simulink library "library"  (R2021a)
settings: Solver=VariableStepAuto  StartTime=0.0  StopTime=10.0  RelTol=1e-3
values from neighbouring files (symbols this model uses):
  sensors = struct()    [setup.m]
  spacecraft = struct()    [setup.m]
undefined symbols (not defined in the file or in its folder): actuators, constants, control, observer, orbit
libraries: vrlib x14, $bdroot x5, cstblocks x1, simulink_extras x1
(part 1 of 2)
settings Model: Creator=loren  LastModifiedBy=loren
settings SolverCC: AlgebraicLoopSolver=TrustRegion
settings DebuggingCC: SFMachineParentedDataDiag=warning

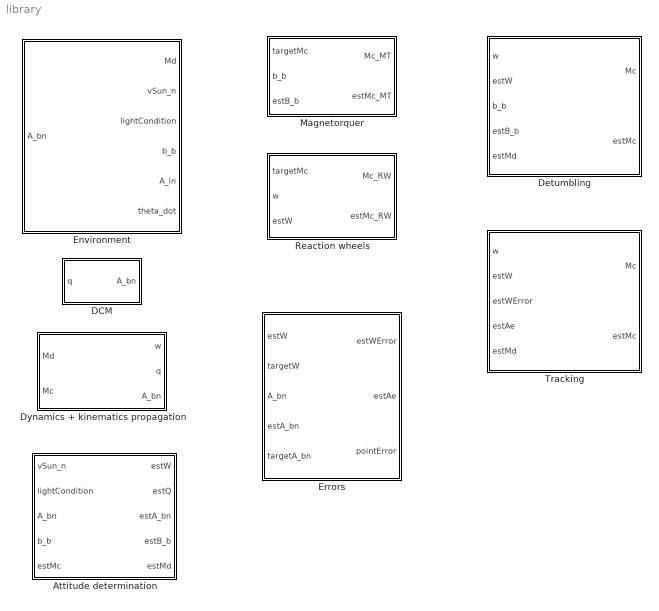
== system library ==
  Attitude determination : Subsystem
  DCM : Subsystem
  Detumbling : Subsystem
  Dynamics + kinematics propagation : Subsystem
  Environment : Subsystem
  Errors : Subsystem
  Magnetorquer : Subsystem
  Reaction wheels : Subsystem
  Tracking : Subsystem

== system library/Attitude determination ==
  vSun_n : Inport
  lightCondition : Inport  Port=2
  A_bn : Inport  Port=3
  b_b : Inport  Port=4
  estMc : Inport  Port=5
  Extended State Observer : Subsystem
  QUEST method : Subsystem
  Sensors : Subsystem
  estW : Outport
  estQ : Outport  Port=2
  estA_bn : Outport  Port=3
  estB_b : Outport  Port=4
  estMd : Outport  Port=5
  wires:
  Sensors/3(sunInSSFoV) -> QUEST method/3(sunInSSFoV)
  Sensors/2(v_n) -> QUEST method/2(v_n)
  Sensors/1(s_b) -> QUEST method/1(s_b)
  vSun_n/1 -> Sensors/1(vSun_n)
  lightCondition/1 -> Sensors/2(lightCondition)
  A_bn/1 -> Sensors/3(A_bn)
  b_b/1 -> Sensors/4(b_b)
  QUEST method/3(quatW) -> Extended State Observer/1(quatW)
  estMc/1 -> Extended State Observer/2(estMc)
  Extended State Observer/1(estW) -> estW/1
  Extended State Observer/2(estMd) -> estMd/1
  QUEST method/2(estA_bn) -> estA_bn/1
  QUEST method/1(estQ) -> estQ/1
  Sensors/4(estB_b) -> estB_b/1

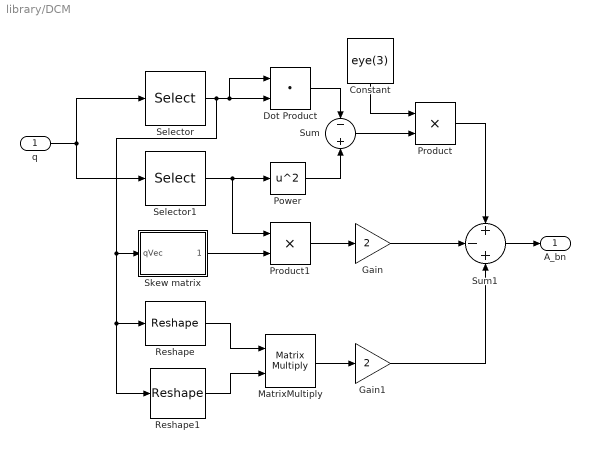
== system library/DCM ==
  q : Inport
  Constant : Constant  Value=eye(3)
  Dot Product : DotProduct  InputSameDT=on  OutDataTypeStr=Inherit: Inherit via internal rule
  Gain : Gain  Gain=2
  Gain1 : Gain  Gain=2
  MatrixMultiply : Product  Multiplication=Matrix(*)
  Power : Math  Operator=square  SaturateOnIntegerOverflow=on
  Product : Product
  Product1 : Product
  Reshape : Reshape  OutputDimensionality=Column vector (2-D)
  Reshape1 : Reshape  OutputDimensionality=Row vector (2-D)
  Selector : Selector  InputPortWidth=4  IndexOptions=Index vector (dialog)  Indices=[1 2 3]  OutputSizes=1
  Selector1 : Selector  InputPortWidth=4  IndexOptions=Index vector (dialog)  Indices=[4]  OutputSizes=1
  Skew matrix : Subsystem
  Sum : Sum  Inputs=-+
  Sum1 : Sum  Inputs=+-+
  A_bn : Outport
  wires:
  q/1 -> Selector/1, Selector1/1
  Selector/1 -> Reshape1/1, Reshape/1, Skew matrix/1(qVec), Dot Product/2, Dot Product/1
  Selector1/1 -> Product1/1, Power/1
  Power/1 -> Sum/2
  Dot Product/1 -> Sum/1
  Constant/1 -> Product/1
  Sum/1 -> Product/2
  Skew matrix/1(qWedge) -> Product1/2
  Product1/1 -> Gain/1
  Reshape/1 -> MatrixMultiply/1
  Reshape1/1 -> MatrixMultiply/2
  MatrixMultiply/1 -> Gain1/1
  Product/1 -> Sum1/1
  Gain/1 -> Sum1/2
  Gain1/1 -> Sum1/3
  Sum1/1 -> A_bn/1

== system library/Detumbling ==
  w : Inport
  estW : Inport  Port=2
  b_b : Inport  Port=3
  estB_b : Inport  Port=4
  estMd : Inport  Port=5
  Constant : Constant  Value=control.detumbling.SRD
  If : If  IfExpression=u1 == 1
  Merge : Merge
  Merge1 : Merge
  Proportional control (RWs) : Subsystem  TreatAsAtomicUnit=on
  Spin rate damping (MT) : Subsystem  TreatAsAtomicUnit=on
  Mc : Outport
  estMc : Outport  Port=2
  wires:
  Constant/1 -> If/1
  Proportional control (RWs)/2(estMc) -> Merge1/2
  Spin rate damping (MT)/2(estMc) -> Merge1/1
  Proportional control (RWs)/1(Mc) -> Merge/2
  Spin rate damping (MT)/1(Mc) -> Merge/1
  Merge/1 -> Mc/1
  Merge1/1 -> estMc/1
  w/1 -> Proportional control (RWs)/1(w)
  estW/1 -> Proportional control (RWs)/2(estW), Spin rate damping (MT)/1(estW)
  b_b/1 -> Spin rate damping (MT)/2(b_b)
  estB_b/1 -> Spin rate damping (MT)/3(estB_b)
  estMd/1 -> Proportional control (RWs)/3(estMd), Spin rate damping (MT)/4(estMd)
  If/1 -> Spin rate damping (MT)/Action
  If/2 -> Proportional control (RWs)/Action

== system library/Dynamics + kinematics propagation ==
  Md : Inport
  Mc : Inport  Port=2
  Euler equations : Subsystem
  Kinematics : Subsystem
  w : Outport
  q : Outport  Port=2
  A_bn : Outport  Port=3
  wires:
  Md/1 -> Euler equations/1(Md)
  Euler equations/1(w) -> w/1, Kinematics/1(w)
  Kinematics/1(q) -> q/1
  Kinematics/2(A_bn) -> A_bn/1
  Mc/1 -> Euler equations/2(Mc)

== system library/Environment ==
  A_bn : Inport
  Disturbances : Subsystem
  Orbit propagator : Subsystem
  Md : Outport
  vSun_n : Outport  Port=2
  lightCondition : Outport  Port=3
  b_b : Outport  Port=4
  A_ln : Outport  Port=5
  theta_dot : Outport  Port=6
  wires:
  A_bn/1 -> Orbit propagator/1(A_bn), Disturbances/1(A_bn)
  Orbit propagator/1(rrSc_n) -> Disturbances/2(rrSc_n)
  Orbit propagator/2(vvSc_n) -> Disturbances/3(vvSc_n)
  Orbit propagator/3(A_bl) -> Disturbances/4(A_bl)
  Disturbances/1(Md) -> Md/1
  Disturbances/2(vSun_n) -> vSun_n/1
  Disturbances/3(lightCondition) -> lightCondition/1
  Disturbances/4(b_b) -> b_b/1
  Orbit propagator/5(theta_dot) -> theta_dot/1
  Orbit propagator/4(A_ln) -> A_ln/1

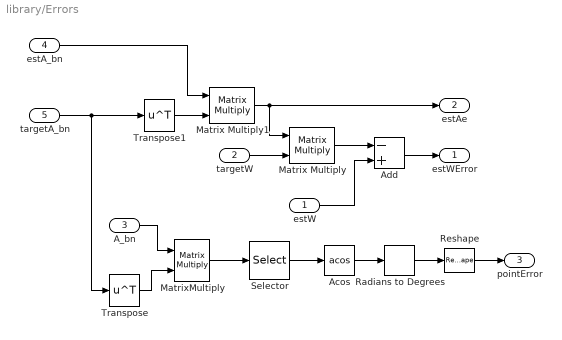
== system library/Errors ==
  estW : Inport
  targetW : Inport  Port=2
  A_bn : Inport  Port=3
  estA_bn : Inport  Port=4
  targetA_bn : Inport  Port=5
  Acos : Trigonometry  Operator=acos
  Add : Sum  Inputs=-+
  Matrix Multiply : Product  Multiplication=Matrix(*)
  Matrix Multiply1 : Product  Multiplication=Matrix(*)
  MatrixMultiply : Product  Multiplication=Matrix(*)
  Radians to Degrees : simulink_extras/Transformations/Radians to Degrees
  Reshape : Reshape
  Selector : Selector  NumberOfDimensions=2  InputPortWidth=3  IndexOptions=Index vector (dialog),Index vector (dialog)  Indices=1,1  OutputSizes=1,1
  Transpose : Math  Operator=transpose  SaturateOnIntegerOverflow=on
  Transpose1 : Math  Operator=transpose  SaturateOnIntegerOverflow=on
  estWError : Outport
  estAe : Outport  Port=2
  pointError : Outport  Port=3
  wires:
  targetW/1 -> Matrix Multiply/2
  targetA_bn/1 -> Transpose/1, Transpose1/1
  estA_bn/1 -> Matrix Multiply1/1
  Matrix Multiply1/1 -> Matrix Multiply/1, estAe/1
  Matrix Multiply/1 -> Add/1
  Acos/1 -> Radians to Degrees/1
  Radians to Degrees/1 -> Reshape/1
  estW/1 -> Add/2
  Add/1 -> estWError/1
  A_bn/1 -> MatrixMultiply/1
  Transpose/1 -> MatrixMultiply/2
  MatrixMultiply/1 -> Selector/1
  Selector/1 -> Acos/1
  Transpose1/1 -> Matrix Multiply1/2
  Reshape/1 -> pointError/1

== system library/Magnetorquer ==
  targetMc : Inport
  b_b : Inport  Port=2
  estB_b : Inport  Port=3
  Cross Product : vrlib/Utilities/Cross Product
  Cross Product1 : vrlib/Utilities/Cross Product
  Cross Product2 : vrlib/Utilities/Cross Product
  Divide : Product  Inputs=/*
  Dot Product : DotProduct  InputSameDT=on  OutDataTypeStr=Inherit: Inherit via internal rule
  Saturation : Saturate  UpperLimit=actuators.mt.D_max  LowerLimit=actuators.mt.D_min
  Mc_MT : Outport
  estMc_MT : Outport  Port=2
  wires:
  b_b/1 -> Cross Product1/2
  Cross Product2/1 -> estMc_MT/1
  Dot Product/1 -> Divide/1
  Cross Product1/1 -> Mc_MT/1
  Saturation/1 -> Cross Product2/1, Cross Product1/1
  targetMc/1 -> Cross Product/2
  Divide/1 -> Saturation/1
  Cross Product/1 -> Divide/2
  estB_b/1 -> Cross Product2/2, Dot Product/1, Dot Product/2, Cross Product/1

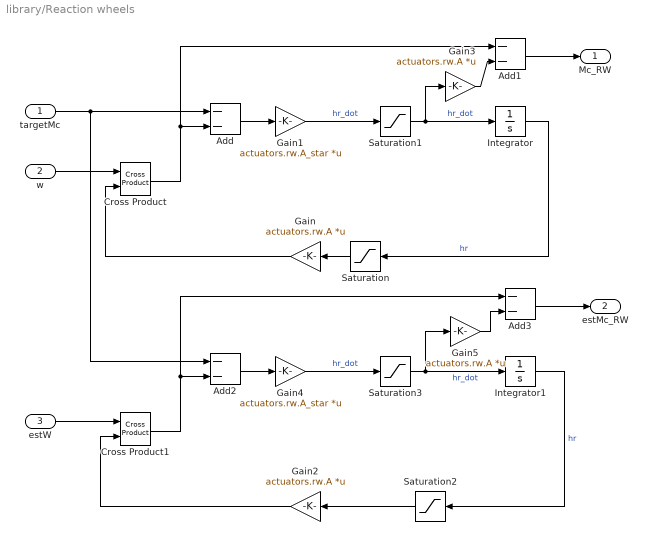
== system library/Reaction wheels ==
  targetMc : Inport
  w : Inport  Port=2
  estW : Inport  Port=3
  Add{,1..3} (4 alike) : Sum  Inputs=--
  Cross Product : vrlib/Utilities/Cross Product
  Cross Product1 : vrlib/Utilities/Cross Product
  Gain{,2..3,5} (4 alike) : Gain  Gain=actuators.rw.A  Multiplication=Matrix(K*u) (u vector)
  Gain1 : Gain  Gain=actuators.rw.A_star  Multiplication=Matrix(K*u) (u vector)
  Gain4 : Gain  Gain=actuators.rw.A_star  Multiplication=Matrix(K*u) (u vector)
  Integrator : Integrator  InitialCondition=actuators.rw.hr0
  Integrator1 : Integrator  InitialCondition=actuators.rw.hr0
  Saturation : Saturate  UpperLimit=actuators.rw.h_max  LowerLimit=-actuators.rw.h_max
  Saturation1 : Saturate  UpperLimit=actuators.rw.hdot_max  LowerLimit=-actuators.rw.hdot_max
  Saturation2 : Saturate  UpperLimit=actuators.rw.h_max  LowerLimit=-actuators.rw.h_max
  Saturation3 : Saturate  UpperLimit=actuators.rw.hdot_max  LowerLimit=-actuators.rw.hdot_max
  Mc_RW : Outport
  estMc_RW : Outport  Port=2
  wires:
  w/1 -> Cross Product/1
  Gain/1 -> Cross Product/2
  Cross Product/1 -> Add/2, Add1/1
  Gain1/1 -> Saturation1/1  "hr_dot"
  Integrator/1 -> Saturation/1  "hr"
  Saturation/1 -> Gain/1
  Add1/1 -> Mc_RW/1
  Add/1 -> Gain1/1
  Gain3/1 -> Add1/2
  Saturation1/1 -> Gain3/1, Integrator/1  "hr_dot"
  Gain5/1 -> Add3/2
  Add3/1 -> estMc_RW/1
  Add2/1 -> Gain4/1
  Saturation3/1 -> Integrator1/1, Gain5/1  "hr_dot"
  Cross Product1/1 -> Add2/2, Add3/1
  Integrator1/1 -> Saturation2/1  "hr"
  estW/1 -> Cross Product1/1
  targetMc/1 -> Add2/1, Add/1
  Saturation2/1 -> Gain2/1
  Gain2/1 -> Cross Product1/2
  Gain4/1 -> Saturation3/1  "hr_dot"

== system library/Tracking ==
  w : Inport
  estW : Inport  Port=2
  estWError : Inport  Port=3
  estAe : Inport  Port=4
  estMd : Inport  Port=5
  Ideal control law : Subsystem
  Reaction wheels : $bdroot/Reaction wheels  SystemSampleTime=-1  VariantActivationTime=update diagram  Latency=0  AutoFrameSizeCalculation=off
  Mc : Outport
  estMc : Outport  Port=2
  wires:
  w/1 -> Reaction wheels/2
  Ideal control law/1(Mc_id) -> Reaction wheels/1
  estW/1 -> Reaction wheels/3, Ideal control law/1(estW)
  estWError/1 -> Ideal control law/2(estWError)
  estAe/1 -> Ideal control law/3(estAe)
  estMd/1 -> Ideal control law/4(estMd)
  Reaction wheels/1 -> Mc/1
  Reaction wheels/2 -> estMc/1

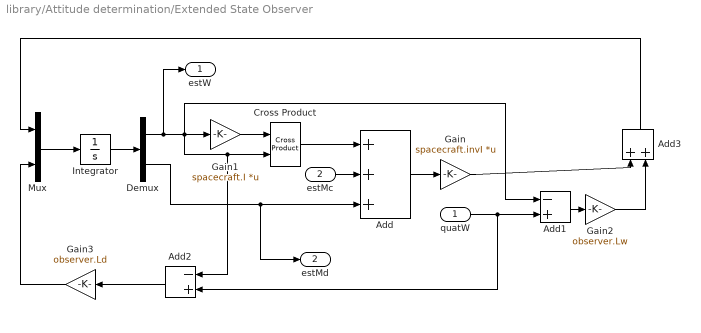
== system library/Attitude determination/Extended State Observer ==
  quatW : Inport
  estMc : Inport  Port=2
  Add : Sum  Inputs=+++
  Add1 : Sum  Inputs=-+
  Add2 : Sum  Inputs=-+
  Add3 : Sum
  Cross Product : vrlib/Utilities/Cross Product
  Demux : Demux  Outputs=[3, 3]
  Gain : Gain  Gain=spacecraft.invI  Multiplication=Matrix(K*u) (u vector)
  Gain1 : Gain  Gain=spacecraft.I  Multiplication=Matrix(K*u) (u vector)
  Gain2 : Gain  Gain=observer.Lw
  Gain3 : Gain  Gain=observer.Ld
  Integrator : Integrator  InitialCondition=[spacecraft.w0; observer.estMd0]
  Mux : Mux  Inputs=[3,3]
  estW : Outport
  estMd : Outport  Port=2
  wires:
  quatW/1 -> Add2/2, Add1/2
  Gain/1 -> Add3/1
  Demux/1 -> Add2/1, Cross Product/2, Add1/1, Gain1/1, estW/1
  Gain1/1 -> Cross Product/1
  Cross Product/1 -> Add/1
  estMc/1 -> Add/2
  Integrator/1 -> Demux/1
  Demux/2 -> estMd/1, Add/3
  Add/1 -> Gain/1
  Add1/1 -> Gain2/1
  Mux/1 -> Integrator/1
  Gain2/1 -> Add3/2
  Add2/1 -> Gain3/1
  Gain3/1 -> Mux/2
  Add3/1 -> Mux/1

== system library/Attitude determination/QUEST method ==
  s_b : Inport
  v_n : Inport  Port=2
  sunInSSFoV : Inport  Port=3
  Angular velocity estimation : Subsystem
  DCM : $bdroot/DCM  SystemSampleTime=-1  VariantActivationTime=update diagram  Latency=0  AutoFrameSizeCalculation=off
  MATLAB Function : MATLAB Function  TreatAsAtomicUnit=on
  Memory : Memory  InitialCondition=spacecraft.q0
  estQ : Outport
  estA_bn : Outport  Port=2
  quatW : Outport  Port=3
  wires:
  s_b/1 -> MATLAB Function/1(s_b)
  v_n/1 -> MATLAB Function/2(v_n)
  sunInSSFoV/1 -> MATLAB Function/3(sunInSSFoV)
  DCM/1 -> estA_bn/1
  Angular velocity estimation/1(quatW) -> quatW/1
  MATLAB Function/1(estQ) -> Memory/1, DCM/1, estQ/1, Angular velocity estimation/1(estQ)
  Memory/1 -> MATLAB Function/4(q_old)

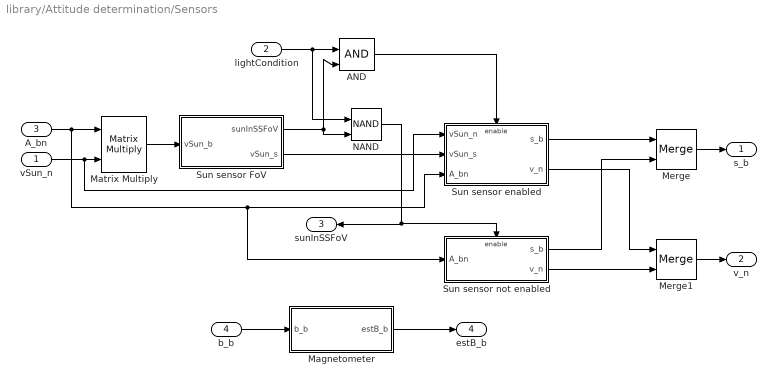
== system library/Attitude determination/Sensors ==
  vSun_n : Inport
  lightCondition : Inport  Port=2
  A_bn : Inport  Port=3
  b_b : Inport  Port=4
  AND : Logic  IconShape=distinctive  AllPortsSameDT=off  OutDataTypeStr=boolean
  Magnetometer : Subsystem
  Matrix Multiply : Product  Multiplication=Matrix(*)
  Merge : Merge
  Merge1 : Merge
  NAND : Logic  Operator=NAND  IconShape=distinctive  AllPortsSameDT=off  OutDataTypeStr=boolean
  Sun sensor FoV : Subsystem
  Sun sensor enabled : Subsystem  TreatAsAtomicUnit=on
  Sun sensor not enabled : Subsystem  TreatAsAtomicUnit=on
  s_b : Outport
  v_n : Outport  Port=2
  sunInSSFoV : Outport  Port=3
  estB_b : Outport  Port=4
  wires:
  Matrix Multiply/1 -> Sun sensor FoV/1(vSun_b)
  vSun_n/1 -> Sun sensor enabled/1(vSun_n), Matrix Multiply/2
  A_bn/1 -> Sun sensor not enabled/1(A_bn), Sun sensor enabled/3(A_bn), Matrix Multiply/1
  Merge/1 -> s_b/1
  Merge1/1 -> v_n/1
  b_b/1 -> Magnetometer/1(b_b)
  Magnetometer/1(estB_b) -> estB_b/1
  lightCondition/1 -> NAND/1, AND/1
  Sun sensor FoV/1(sunInSSFoV) -> AND/2, NAND/2
  AND/1 -> Sun sensor enabled/Enable
  NAND/1 -> sunInSSFoV/1, Sun sensor not enabled/Enable
  Sun sensor FoV/2(vSun_s) -> Sun sensor enabled/2(vSun_s)
  Sun sensor enabled/1(s_b) -> Merge/1
  Sun sensor not enabled/1(s_b) -> Merge/2
  Sun sensor enabled/2(v_n) -> Merge1/1
  Sun sensor not enabled/2(v_n) -> Merge1/2

== system library/DCM/Skew matrix ==
  qVec : Inport
  Constant : Constant  Value=0
  Constant1 : Constant  Value=0
  Constant2 : Constant  Value=0
  Demux : Demux  Outputs=3
  Gain : Gain  Gain=-1
  Gain1 : Gain  Gain=-1
  Gain2 : Gain  Gain=-1
  Matrix Concatenate : Concatenate  NumInputs=3  Mode=Multidimensional array
  Mux : Mux  Inputs=3
  Mux1 : Mux  Inputs=3
  Mux2 : Mux  Inputs=3
  Reshape : Reshape  OutputDimensionality=Row vector (2-D)
  Reshape1 : Reshape  OutputDimensionality=Row vector (2-D)
  Reshape2 : Reshape  OutputDimensionality=Row vector (2-D)
  qWedge : Outport
  wires:
  qVec/1 -> Demux/1
  Constant/1 -> Mux/1
  Gain/1 -> Mux/2
  Demux/3 -> Mux1/1, Gain/1
  Demux/2 -> Gain2/1, Mux/3
  Constant1/1 -> Mux1/2
  Gain1/1 -> Mux1/3
  Demux/1 -> Mux2/2, Gain1/1
  Constant2/1 -> Mux2/3
  Gain2/1 -> Mux2/1
  Mux1/1 -> Reshape1/1
  Mux/1 -> Reshape/1
  Mux2/1 -> Reshape2/1
  Matrix Concatenate/1 -> qWedge/1
  Reshape/1 -> Matrix Concatenate/1
  Reshape1/1 -> Matrix Concatenate/2
  Reshape2/1 -> Matrix Concatenate/3

== system library/Detumbling/Proportional control (RWs) ==
  w : Inport
  estW : Inport  Port=2
  estMd : Inport  Port=3
  Action Port : ActionPort
  Ideal control law : Subsystem  TreatAsAtomicUnit=on
  Reaction wheels : $bdroot/Reaction wheels  SystemSampleTime=-1  VariantActivationTime=update diagram  Latency=0  AutoFrameSizeCalculation=off
  Mc : Outport
  estMc : Outport  Port=2
  wires:
  Reaction wheels/1 -> Mc/1
  estMd/1 -> Ideal control law/2(estMd)
  estW/1 -> Ideal control law/1(estW), Reaction wheels/3
  w/1 -> Reaction wheels/2
  Ideal control law/1(Mc_id) -> Reaction wheels/1
  Reaction wheels/2 -> estMc/1

== system library/Detumbling/Spin rate damping (MT) ==
  estW : Inport
  b_b : Inport  Port=2
  estB_b : Inport  Port=3
  estMd : Inport  Port=4
  Action Port : ActionPort
  Ideal control law : Subsystem
  Magnetorquer : $bdroot/Magnetorquer  SystemSampleTime=-1  VariantActivationTime=update diagram  Latency=0  AutoFrameSizeCalculation=off
  Mc : Outport
  estMc : Outport  Port=2
  wires:
  Magnetorquer/2 -> estMc/1
  estW/1 -> Ideal control law/1(estW)
  estMd/1 -> Ideal control law/3(estMd)
  Magnetorquer/1 -> Mc/1
  Ideal control law/1(targetMc) -> Magnetorquer/1
  estB_b/1 -> Magnetorquer/3, Ideal control law/2(estB_b)
  b_b/1 -> Magnetorquer/2

== system library/Dynamics + kinematics propagation/Euler equations ==
  Md : Inport
  Mc : Inport  Port=2
  Add : Sum  Inputs=+++
  Cross Product : vrlib/Utilities/Cross Product
  Gain : Gain  Gain=spacecraft.I  Multiplication=Matrix(K*u) (u vector)
  Gain1 : Gain  Gain=spacecraft.invI  Multiplication=Matrix(K*u) (u vector)
  Integrator : Integrator  InitialCondition=spacecraft.w0
  w : Outport
  wires:
  Gain/1 -> Cross Product/1
  Integrator/1 -> w/1, Cross Product/2, Gain/1
  Cross Product/1 -> Add/1
  Gain1/1 -> Integrator/1
  Add/1 -> Gain1/1
  Md/1 -> Add/2
  Mc/1 -> Add/3

== system library/Dynamics + kinematics propagation/Kinematics ==
  w : Inport
  DCM : $bdroot/DCM  SystemSampleTime=-1  VariantActivationTime=update diagram  Latency=0  AutoFrameSizeCalculation=off
  Quaternion integration : Subsystem
  q : Outport
  A_bn : Outport  Port=2
  wires:
  w/1 -> Quaternion integration/1(w)
  Quaternion integration/1(q) -> DCM/1, q/1
  DCM/1 -> A_bn/1

== system library/Environment/Disturbances ==
  A_bn : Inport
  rrSc_n : Inport  Port=2
  vvSc_n : Inport  Port=3
  A_bl : Inport  Port=4
  Drag : Subsystem
  Earth magnetic field : Subsystem
  Gravity gradient : Subsystem
  Solar radiation pressure : Subsystem
      settings: PortSchema="{\"entries\":[{\"content\":{\"sides\":[{\"content\":{\"connectorIds\":[\"In1\",\"In2\"]},\"type\":\"ConnectorPlacement.EquallySpacedRectSide\",\"uuid\":\"1c58e148-737e-4c26-8467-bf4a1427bac3\"},{\"content\":{\"connectorIds\":[\"Out1\"],\"side\":\"RIGHT\"},\"type\":\"ConnectorPlacement.EquallySpacedRectSide\",\"uuid\":\"1132a1c1-392d-4550-8b40-4ae647f3a6c1\"},{\"content\":{\"connectorIds\":[\"Out2\",\"Out3\"],\"side\":\"TOP\"},\"type\":\"ConnectorPlacement.EquallySpacedRectSide\",\"uuid\":\"8cec875a-7b2b-408d-843f-f50e353248f2\"},{\"content\":{\"connectorIds\":[],\"side\":\"HIDDEN\"},\"type\":\"ConnectorPlacement.EquallySpacedRectSide\",\"uuid\":\"95559ba3-4215-4144-a5e7-008848b1ca72\"}]},\"type\":\"ConnectorPlacement.EquallySpacedConnector\",\"uuid\":\"cb15f690-b6d7-424c-84c7-df23a46a4e4f\"}],\"packageUris\":[\"http://schema.mathworks.com/mf0/Connector/R2020b\"],\"version\":\"1.0\"}"
  Sum : Sum  Inputs=++++
  Md : Outport
  vSun_n : Outport  Port=2
  lightCondition : Outport  Port=3
  b_b : Outport  Port=4
  wires:
  Solar radiation pressure/1(M_srp) -> Sum/1
  A_bn/1 -> Solar radiation pressure/2(A_bn), Drag/3(A_bn), Earth magnetic field/2(A_bn)
  vvSc_n/1 -> Drag/2(vvSc_n)
  rrSc_n/1 -> Gravity gradient/1(rrSc_n), Drag/1(rrSc_n), Earth magnetic field/1(rrSc_n), Solar radiation pressure/1(rrSc_n)
  Gravity gradient/1(M_gg) -> Sum/3
  Drag/1(M_drag) -> Sum/4
  Earth magnetic field/2(M_b) -> Sum/2
  Sum/1 -> Md/1
  A_bl/1 -> Gravity gradient/2(A_bl)
  Solar radiation pressure/2(vSun_n) -> vSun_n/1
  Solar radiation pressure/3(lightCondition) -> lightCondition/1
  Earth magnetic field/1(b_b) -> b_b/1

== system library/Environment/Orbit propagator ==
  A_bn : Inport
  Integrator1 : Integrator  InitialCondition=orbit.theta0
  LVLH frame : Subsystem
  Position and velocity (inertial frame) : Subsystem
  True anomaly ODE : Subsystem
  rrSc_n : Outport
  vvSc_n : Outport  Port=2
  A_bl : Outport  Port=3
  A_ln : Outport  Port=4
  theta_dot : Outport  Port=5
  wires:
  True anomaly ODE/1(theta_dot) -> Integrator1/1, theta_dot/1
  Integrator1/1 -> LVLH frame/1(theta), True anomaly ODE/1(theta), Position and velocity (inertial frame)/1(theta)
  Position and velocity (inertial frame)/1(rrSc_n) -> rrSc_n/1
  Position and velocity (inertial frame)/2(vvSc_n) -> vvSc_n/1
  LVLH frame/1(A_bl) -> A_bl/1
  A_bn/1 -> LVLH frame/2(A_bn)
  LVLH frame/2(A_ln) -> A_ln/1

== system library/Tracking/Ideal control law ==
  estW : Inport
  estWError : Inport  Port=2
  estAe : Inport  Port=3
  estMd : Inport  Port=4
  Add : Sum  Inputs=--+-
  Cross Product : vrlib/Utilities/Cross Product
  Gain : Gain  Gain=control.tracking.kw
  Gain1 : Gain  Gain=control.tracking.kae
  Gain3 : Gain  Gain=spacecraft.I  Multiplication=Matrix(K*u) (u vector)
  MATLAB Function : MATLAB Function  TreatAsAtomicUnit=on
  Mc_id : Outport
  wires:
  Add/1 -> Mc_id/1
  MATLAB Function/1(lf) -> Gain1/1
  estAe/1 -> MATLAB Function/1(estAe)
  Gain/1 -> Add/1
  Gain3/1 -> Cross Product/2
  estMd/1 -> Add/4
  Gain1/1 -> Add/2
  estWError/1 -> Gain/1
  estW/1 -> Gain3/1, Cross Product/1
  Cross Product/1 -> Add/3

== system library/Attitude determination/QUEST method/Angular velocity estimation ==
  estQ : Inport
  Constant : Constant
  Derivative : Derivative  CoefficientInTFapproximation=1/10
  Gain : Gain  Gain=2
  Matrix Multiply : Product  Multiplication=Matrix(*)
  Quaternion matrix : Subsystem
  Varying Lowpass Filter : cstblocks/Linear Parameter Varying/Varying Lowpass Filter  N=1
  quatW : Outport
  wires:
  Derivative/1 -> Matrix Multiply/2  "dotQest"
  Matrix Multiply/1 -> Gain/1
  Gain/1 -> quatW/1
  estQ/1 -> Quaternion matrix/1(q), Varying Lowpass Filter/1
  Varying Lowpass Filter/1 -> Derivative/1
  Constant/1 -> Varying Lowpass Filter/2
  Quaternion matrix/1(Q_star) -> Matrix Multiply/1

== system library/Attitude determination/Sensors/Magnetometer ==
  b_b : Inport
  Add : Sum
  MATLAB Function : MATLAB Function  TreatAsAtomicUnit=on
  Matrix Multiply : Product  Multiplication=Matrix(*)
  Random Number : RandomNumber  Variance=sensors.mm.sigmaPhi^2  Seed=randi(1e5, 1, 1)  SampleTime=sensors.mm.Ts
  Random Number1 : RandomNumber  Variance=sensors.mm.sigmaTheta^2  Seed=randi(1e5, 1, 1)  SampleTime=sensors.mm.Ts
  Random Number2 : RandomNumber  Variance=sensors.mm.sigmaPsi^2  Seed=randi(1e5, 1, 1)  SampleTime=sensors.mm.Ts
  Random Number3 : RandomNumber  Variance=sensors.mm.eps^2*ones(3,1)  Seed=randi(1e5, 1, 1)  SampleTime=sensors.mm.Ts
  Zero-Order Hold : ZeroOrderHold  SampleTime=sensors.mm.Ts
  estB_b : Outport
  wires:
  b_b/1 -> Zero-Order Hold/1
  Random Number/1 -> MATLAB Function/1(phi)
  Random Number1/1 -> MATLAB Function/2(theta)
  Random Number2/1 -> MATLAB Function/3(psi)
  Zero-Order Hold/1 -> Add/1
  MATLAB Function/1(A_err) -> Matrix Multiply/1
  Matrix Multiply/1 -> estB_b/1
  Add/1 -> Matrix Multiply/2
  Random Number3/1 -> Add/2

== system library/Attitude determination/Sensors/Sun sensor FoV ==
  vSun_b : Inport
  Acos : Trigonometry  Operator=acos
  Constant : Constant  Value=sensors.ss.FoV
  Constant2 : Constant  Value=[1; 0; 0]
  Dot Product : DotProduct  InputSameDT=on  OutDataTypeStr=Inherit: Inherit via internal rule
  Gain : Gain  Gain=sensors.ss.A_sb  Multiplication=Matrix(K*u) (u vector)
  Less Than : RelationalOperator  Operator=<  OutDataTypeStr=boolean  RndMeth=Simplest
  sunInSSFoV : Outport
  vSun_s : Outport  Port=2
  wires:
  Less Than/1 -> sunInSSFoV/1
  Constant/1 -> Less Than/2
  Acos/1 -> Less Than/1
  Dot Product/1 -> Acos/1
  vSun_b/1 -> Gain/1
  Gain/1 -> Dot Product/2, vSun_s/1
  Constant2/1 -> Dot Product/1

== system library/Attitude determination/Sensors/Sun sensor enabled ==
  vSun_n : Inport
  vSun_s : Inport  Port=2
  A_bn : Inport  Port=3
  Enable : EnablePort
  Matrix Concatenate : Concatenate  Mode=Multidimensional array  ConcatenateDimension=2
  Matrix Concatenate1 : Concatenate  Mode=Multidimensional array  ConcatenateDimension=2
  Star tracker : Subsystem
  Sun sensor : Subsystem
  Zero-Order Hold : ZeroOrderHold  SampleTime=max([sensors.ss.Ts, sensors.st.Ts])
  s_b : Outport
  v_n : Outport  Port=2
  wires:
  vSun_s/1 -> Sun sensor/1(vSun_s)
  A_bn/1 -> Star tracker/1(A_bn)
  Sun sensor/1(sSun_b) -> Matrix Concatenate/1
  Star tracker/1(sStars_b) -> Matrix Concatenate/2
  Star tracker/2(vStars_n) -> Matrix Concatenate1/2
  vSun_n/1 -> Zero-Order Hold/1
  Matrix Concatenate/1 -> s_b/1
  Matrix Concatenate1/1 -> v_n/1
  Zero-Order Hold/1 -> Matrix Concatenate1/1

== system library/Attitude determination/Sensors/Sun sensor not enabled ==
  A_bn : Inport
  Enable : EnablePort
  Star tracker : Subsystem
  s_b : Outport
  v_n : Outport  Port=2
  wires:
  Star tracker/1(sStars_b) -> s_b/1
  Star tracker/2(vStars_n) -> v_n/1
  A_bn/1 -> Star tracker/1(A_bn)

== system library/Detumbling/Proportional control (RWs)/Ideal control law ==
  estW : Inport
  estMd : Inport  Port=2
  Add : Sum  Inputs=+-
  Gain : Gain  Gain=-control.detumbling.kp
  Mc_id : Outport
  wires:
  estMd/1 -> Add/2
  Add/1 -> Mc_id/1
  Gain/1 -> Add/1
  estW/1 -> Gain/1

== system library/Detumbling/Spin rate damping (MT)/Ideal control law ==
  estW : Inport
  estB_b : Inport  Port=2
  estMd : Inport  Port=3
  Add : Sum  Inputs=+-
  Cross Product : vrlib/Utilities/Cross Product
  Cross Product1 : vrlib/Utilities/Cross Product
  Gain : Gain  Gain=-control.detumbling.kb
  targetMc : Outport
  wires:
  Cross Product1/1 -> Add/1
  Gain/1 -> Cross Product1/1
  estW/1 -> Cross Product/2
  estB_b/1 -> Cross Product1/2, Cross Product/1
  Cross Product/1 -> Gain/1
  Add/1 -> targetMc/1
  estMd/1 -> Add/2

== system library/Dynamics + kinematics propagation/Kinematics/Quaternion integration ==
  w : Inport
  Gain : Gain  Gain=1/2
  Integrator : Integrator  InitialCondition=spacecraft.q0
  MatrixMultiply : Product  Multiplication=Matrix(*)
  Normalize Vector : vrlib/Utilities/Normalize Vector  maxzero=0
  Omega matrix : Subsystem
  q : Outport
  wires:
  Integrator/1 -> Normalize Vector/1
  Normalize Vector/1 -> q/1, MatrixMultiply/2
  Omega matrix/1(OM_mat) -> MatrixMultiply/1
  MatrixMultiply/1 -> Gain/1
  Gain/1 -> Integrator/1
  w/1 -> Omega matrix/1(w)

== system library/Environment/Disturbances/Drag ==
  rrSc_n : Inport
  vvSc_n : Inport  Port=2
  A_bn : Inport  Port=3
  Constant : Constant  Value=constants.rho
  MATLAB Function : MATLAB Function  TreatAsAtomicUnit=on
  M_drag : Outport
  wires:
  rrSc_n/1 -> MATLAB Function/1(rrSc_n)
  MATLAB Function/1(mDrag) -> M_drag/1
  vvSc_n/1 -> MATLAB Function/2(vvSc_n)
  A_bn/1 -> MATLAB Function/3(A_bn)
  Constant/1 -> MATLAB Function/4(rho)

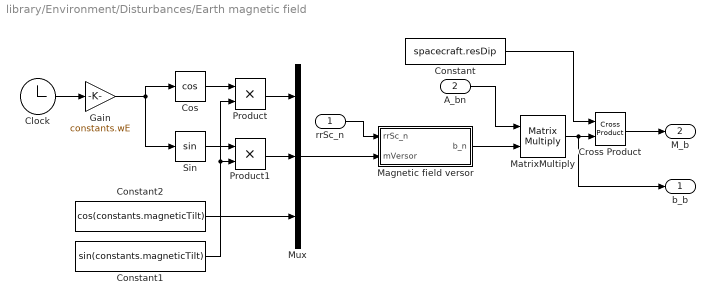
== system library/Environment/Disturbances/Earth magnetic field ==
  rrSc_n : Inport
  A_bn : Inport  Port=2
  Clock : Clock
  Constant : Constant  Value=spacecraft.resDip
  Constant1 : Constant  Value=sin(constants.magneticTilt)
  Constant2 : Constant  Value=cos(constants.magneticTilt)
  Cos : Trigonometry  Operator=cos
  Cross Product : vrlib/Utilities/Cross Product
  Gain : Gain  Gain=constants.wE
  Magnetic field versor : Subsystem
  MatrixMultiply : Product  Multiplication=Matrix(*)
  Mux : Mux  Inputs=3
  Product : Product
  Product1 : Product
  Sin : Trigonometry
  b_b : Outport
  M_b : Outport  Port=2
  wires:
  Clock/1 -> Gain/1
  Constant/1 -> Cross Product/1
  Gain/1 -> Sin/1, Cos/1
  Constant2/1 -> Mux/3
  Sin/1 -> Product1/1
  Cos/1 -> Product/1
  Product/1 -> Mux/1
  Product1/1 -> Mux/2
  Constant1/1 -> Product/2, Product1/2
  A_bn/1 -> MatrixMultiply/1
  rrSc_n/1 -> Magnetic field versor/1(rrSc_n)
  Mux/1 -> Magnetic field versor/2(mVersor)
  Magnetic field versor/1(b_n) -> MatrixMultiply/2
  MatrixMultiply/1 -> b_b/1, Cross Product/2
  Cross Product/1 -> M_b/1

== system library/Environment/Disturbances/Gravity gradient ==
  rrSc_n : Inport
  A_bl : Inport  Port=2
  Constant : Constant  Value=[1 0 0]
  Gravity gradient : Subsystem
  MatrixMultiply : Product  Multiplication=Matrix(*)
  M_gg : Outport
  wires:
  Constant/1 -> MatrixMultiply/2
  MatrixMultiply/1 -> Gravity gradient/2(c)  "c"
  A_bl/1 -> MatrixMultiply/1
  Gravity gradient/1(M_gg) -> M_gg/1
  rrSc_n/1 -> Gravity gradient/1(rrSc_n)

== system library/Environment/Disturbances/Solar radiation pressure ==
  note: Determine whether the s/c is in sunlight or not
  rrSc_n : Inport
  A_bn : Inport  Port=2
  If : If  IfExpression=u1 == 1
  Merge : Merge
  SRP: active : Subsystem  TreatAsAtomicUnit=on
  SRP: non-active : Subsystem  TreatAsAtomicUnit=on
  Shadow cone of the Earth : Subsystem
  Sun position in the Earth inertial frame : Subsystem
  M_srp : Outport
  vSun_n : Outport  Port=2
  lightCondition : Outport  Port=3
  wires:
  Shadow cone of the Earth/1(lightCondition) -> lightCondition/1, If/1
  If/2 -> SRP: non-active/Action
  If/1 -> SRP: active/Action
  SRP: non-active/1(mSRP) -> Merge/2
  rrSc_n/1 -> SRP: active/1(rrSc_n), Shadow cone of the Earth/1(rrSc_n)
  Merge/1 -> M_srp/1
  SRP: active/1(mSRP) -> Merge/1
  Sun position in the Earth inertial frame/1(rrSun_n) -> SRP: active/2(rrSun_n), Shadow cone of the Earth/2(rrSun_n)
  SRP: active/2(vSun_n) -> vSun_n/1
  A_bn/1 -> SRP: active/3(A_bn)

== system library/Environment/Orbit propagator/LVLH frame ==
  theta : Inport
  A_bn : Inport  Port=2
  LVLH to inclined orbit frame : Subsystem
  Product : Product  Multiplication=Matrix(*)
  Product1 : Product  Multiplication=Matrix(*)
  R1(i) : Constant  Value=[1 0 0; 0 cos(orbit.i) sin(orbit.i); 0 -sin(orbit.i) cos(orbit.i)];
  Transpose : Math  Operator=transpose  SaturateOnIntegerOverflow=on
  A_bl : Outport
  A_ln : Outport  Port=2
  wires:
  Transpose/1 -> Product1/2  "A_nl"
  Product/1 -> A_ln/1, Transpose/1
  A_bn/1 -> Product1/1
  Product1/1 -> A_bl/1  "A_bl"
  R1(i)/1 -> Product/2
  theta/1 -> LVLH to inclined orbit frame/1(theta)
  LVLH to inclined orbit frame/1(A_li) -> Product/1

== system library/Environment/Orbit propagator/Position and velocity (inertial frame) ==
  theta : Inport
  Matrix Multiply : Product  Multiplication=Matrix(*)
  Matrix Multiply1 : Product  Multiplication=Matrix(*)
  Position and velocity (perifocal frame) : Subsystem
  R1(i) : Constant  Value=[1 0 0; 0 cos(orbit.i) sin(orbit.i); 0 -sin(orbit.i) cos(orbit.i)];
  R3(OM) : Constant  Value=[cos(orbit.OM), sin(orbit.OM), 0; -sin(orbit.OM), cos(orbit.OM), 0; 0, 0, 1]
  R3(om) : Constant  Value=[cos(orbit.om), sin(orbit.om), 0; -sin(orbit.om), cos(orbit.om), 0; 0, 0, 1]
  Rotation matrix (perifocal-inertial) : Product  Inputs=3  Multiplication=Matrix(*)
  Transpose : Math  Operator=transpose  SaturateOnIntegerOverflow=on
  rrSc_n : Outport
  vvSc_n : Outport  Port=2
  wires:
  Matrix Multiply/1 -> rrSc_n/1
  Position and velocity (perifocal frame)/2(vvSc_pf) -> Matrix Multiply1/2
  Matrix Multiply1/1 -> vvSc_n/1
  R3(om)/1 -> Rotation matrix (perifocal-inertial)/1
  R1(i)/1 -> Rotation matrix (perifocal-inertial)/2
  Rotation matrix (perifocal-inertial)/1 -> Transpose/1
  Transpose/1 -> Matrix Multiply1/1, Matrix Multiply/1
  R3(OM)/1 -> Rotation matrix (perifocal-inertial)/3
  Position and velocity (perifocal frame)/1(rrSc_pf) -> Matrix Multiply/2
  theta/1 -> Position and velocity (perifocal frame)/1(theta)

== system library/Environment/Orbit propagator/True anomaly ODE ==
  theta : Inport
  Add : Sum
  Constant1 : Constant
  Cos : Trigonometry  Operator=cos
  Gain : Gain  Gain=sqrt(constants.mu/orbit.a^3)
  Gain1 : Gain  Gain=(1 - orbit.e^2)^(-3/2)
  Gain2 : Gain  Gain=orbit.e
  Power : Math  Operator=square  SaturateOnIntegerOverflow=on
  theta_dot : Outport
  wires:
  theta/1 -> Cos/1
  Constant1/1 -> Add/1
  Cos/1 -> Gain2/1
  Gain2/1 -> Add/2
  Add/1 -> Power/1
  Power/1 -> Gain/1
  Gain/1 -> Gain1/1
  Gain1/1 -> theta_dot/1

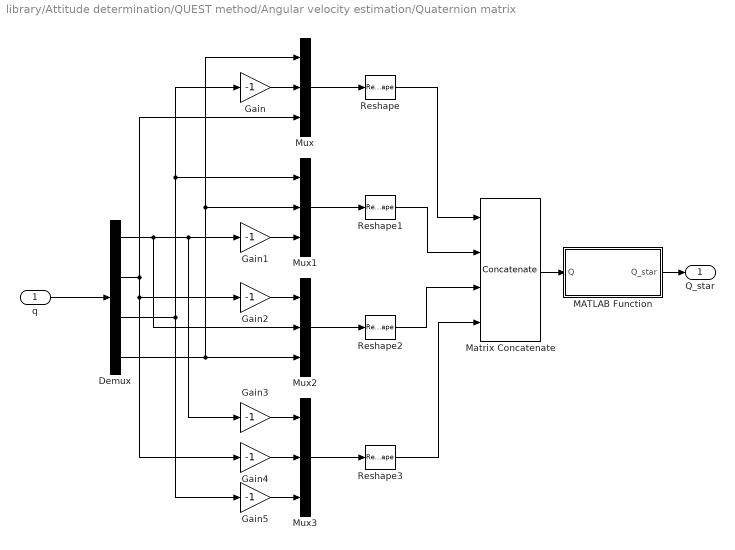
== system library/Attitude determination/QUEST method/Angular velocity estimation/Quaternion matrix ==
  q : Inport
  Demux : Demux
  Gain{,1..5} (6 alike) : Gain  Gain=-1
  MATLAB Function : MATLAB Function  TreatAsAtomicUnit=on
  Matrix Concatenate : Concatenate  NumInputs=4  Mode=Multidimensional array
  Mux{,1..3} (4 alike) : Mux  Inputs=3
  Reshape{,1..3} (4 alike) : Reshape  OutputDimensionality=Row vector (2-D)
  Q_star : Outport
  wires:
  q/1 -> Demux/1
  Demux/4 -> Mux1/2, Mux/1, Mux2/3
  Gain/1 -> Mux/2
  Demux/3 -> Gain5/1, Mux1/1, Gain/1
  Demux/2 -> Gain2/1, Gain4/1, Mux/3
  Gain1/1 -> Mux1/3
  Demux/1 -> Mux2/2, Gain3/1, Gain1/1
  Gain2/1 -> Mux2/1
  Gain3/1 -> Mux3/1
  Gain4/1 -> Mux3/2
  Gain5/1 -> Mux3/3
  Mux3/1 -> Reshape3/1
  Mux2/1 -> Reshape2/1
  Mux1/1 -> Reshape1/1
  Mux/1 -> Reshape/1
  Reshape/1 -> Matrix Concatenate/1
  Reshape1/1 -> Matrix Concatenate/2
  Reshape2/1 -> Matrix Concatenate/3
  Reshape3/1 -> Matrix Concatenate/4
  Matrix Concatenate/1 -> MATLAB Function/1(Q)
  MATLAB Function/1(Q_star) -> Q_star/1

== system library/Attitude determination/Sensors/Sun sensor enabled/Star tracker ==
  A_bn : Inport
  MATLAB Function : MATLAB Function  TreatAsAtomicUnit=on
  Memory : Memory  InitialCondition=sensors.st.vStars_n_init(:,2:end)  InheritSampleTime=on  LinearizeMemory=on
  Random Number : RandomNumber  Variance=sensors.st.sigmaPhi^2  Seed=randi(1e5,1,1)  SampleTime=max([sensors.ss.Ts, sensors.st.Ts])
  Random Number1 : RandomNumber  Variance=sensors.st.sigmaTheta^2  Seed=randi(1e5,1,1)  SampleTime=max([sensors.ss.Ts, sensors.st.Ts])
  Random Number2 : RandomNumber  Variance=sensors.st.sigmaPsi^2  Seed=randi(1e5,1,1)  SampleTime=max([sensors.ss.Ts, sensors.st.Ts])
  Zero-Order Hold : ZeroOrderHold  SampleTime=max([sensors.ss.Ts, sensors.st.Ts])
  sStars_b : Outport
  vStars_n : Outport  Port=2
  wires:
  MATLAB Function/2(v_n) -> Memory/1, vStars_n/1
  MATLAB Function/1(s_b) -> sStars_b/1
  Random Number1/1 -> MATLAB Function/3(theta)
  A_bn/1 -> Zero-Order Hold/1
  Random Number2/1 -> MATLAB Function/4(psi)
  Random Number/1 -> MATLAB Function/2(phi)
  Zero-Order Hold/1 -> MATLAB Function/1(A_bn)
  Memory/1 -> MATLAB Function/5(v_n_old)

== system library/Attitude determination/Sensors/Sun sensor enabled/Sun sensor ==
  vSun_s : Inport
  Gain : Gain  Gain=sensors.ss.A_sb'  Multiplication=Matrix(K*u) (u vector)
  MATLAB Function : MATLAB Function  TreatAsAtomicUnit=on
  MatrixMultiply1 : Product  Multiplication=Matrix(*)
  Random Number : RandomNumber  Variance=sensors.ss.sigmaPhi^2  Seed=randi(1e5, 1, 1)  SampleTime=max([sensors.ss.Ts, sensors.st.Ts])
  Random Number1 : RandomNumber  Variance=sensors.ss.sigmaTheta^2  Seed=randi(1e5, 1, 1)  SampleTime=max([sensors.ss.Ts, sensors.st.Ts])
  Random Number2 : RandomNumber  Variance=sensors.ss.sigmaPsi^2  Seed=randi(1e5, 1, 1)  SampleTime=max([sensors.ss.Ts, sensors.st.Ts])
  Zero-Order Hold : ZeroOrderHold  SampleTime=max([sensors.ss.Ts, sensors.st.Ts])
  sSun_b : Outport
  wires:
  Random Number/1 -> MATLAB Function/1(phi)
  Random Number1/1 -> MATLAB Function/2(theta)
  MATLAB Function/1(A_err) -> MatrixMultiply1/1
  MatrixMultiply1/1 -> Gain/1
  Random Number2/1 -> MATLAB Function/3(psi)
  vSun_s/1 -> Zero-Order Hold/1  "vSun_s"
  Zero-Order Hold/1 -> MatrixMultiply1/2
  Gain/1 -> sSun_b/1

== system library/Attitude determination/Sensors/Sun sensor not enabled/Star tracker ==
  A_bn : Inport
  MATLAB Function : MATLAB Function  TreatAsAtomicUnit=on
  Memory : Memory  InitialCondition=sensors.st.vStars_n_init  InheritSampleTime=on  LinearizeMemory=on
  Random Number : RandomNumber  Variance=sensors.st.sigmaPhi^2  Seed=randi(1e5,1,1)  SampleTime=max([sensors.ss.Ts, sensors.st.Ts])
  Random Number1 : RandomNumber  Variance=sensors.st.sigmaTheta^2  Seed=randi(1e5,1,1)  SampleTime=max([sensors.ss.Ts, sensors.st.Ts])
  Random Number2 : RandomNumber  Variance=sensors.st.sigmaPsi^2  Seed=randi(1e5,1,1)  SampleTime=max([sensors.ss.Ts, sensors.st.Ts])
  Zero-Order Hold : ZeroOrderHold  SampleTime=max([sensors.ss.Ts, sensors.st.Ts])
  sStars_b : Outport
  vStars_n : Outport  Port=2
  wires:
  Memory/1 -> MATLAB Function/5(v_n_old)
  Zero-Order Hold/1 -> MATLAB Function/1(A_bn)
  Random Number/1 -> MATLAB Function/2(phi)
  Random Number2/1 -> MATLAB Function/4(psi)
  A_bn/1 -> Zero-Order Hold/1
  Random Number1/1 -> MATLAB Function/3(theta)
  MATLAB Function/1(s_b) -> sStars_b/1
  MATLAB Function/2(v_n) -> Memory/1, vStars_n/1

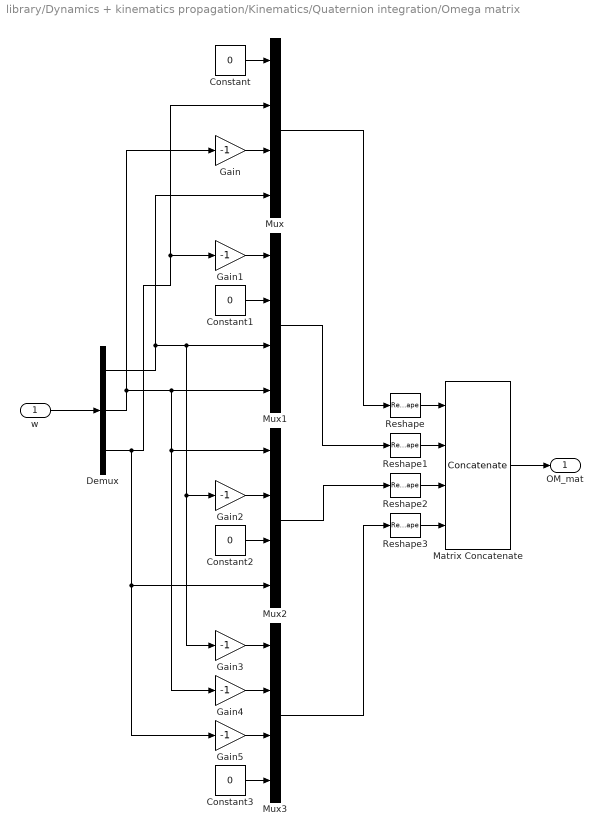
== system library/Dynamics + kinematics propagation/Kinematics/Quaternion integration/Omega matrix ==
  w : Inport
  Constant{,1..3} (4 alike) : Constant  Value=0
  Demux : Demux  Outputs=3
  Gain{,1..5} (6 alike) : Gain  Gain=-1
  Matrix Concatenate : Concatenate  NumInputs=4  Mode=Multidimensional array
  Mux{,1..3} (4 alike) : Mux
  Reshape{,1..3} (4 alike) : Reshape  OutputDimensionality=Row vector (2-D)
  OM_mat : Outport
  wires:
  w/1 -> Demux/1
  Demux/1 -> Mux/4, Gain3/1, Gain2/1, Mux1/3
  Demux/2 -> Gain/1, Mux2/1, Gain4/1, Mux1/4
  Gain/1 -> Mux/3
  Demux/3 -> Mux/2, Gain1/1, Mux2/4, Gain5/1
  Constant/1 -> Mux/1
  Gain1/1 -> Mux1/1
  Constant1/1 -> Mux1/2
  Gain2/1 -> Mux2/2
  Constant2/1 -> Mux2/3
  Gain3/1 -> Mux3/1
  Gain4/1 -> Mux3/2
  Constant3/1 -> Mux3/4
  Gain5/1 -> Mux3/3
  Mux/1 -> Reshape/1
  Mux1/1 -> Reshape1/1
  Mux2/1 -> Reshape2/1
  Mux3/1 -> Reshape3/1
  Matrix Concatenate/1 -> OM_mat/1
  Reshape/1 -> Matrix Concatenate/1
  Reshape1/1 -> Matrix Concatenate/2
  Reshape2/1 -> Matrix Concatenate/3
  Reshape3/1 -> Matrix Concatenate/4

== system library/Environment/Disturbances/Earth magnetic field/Magnetic field versor ==
  rrSc_n : Inport
  mVersor : Inport  Port=2
  Constant : Constant  Value=-3
  Dot Product : DotProduct  InputSameDT=on  OutDataTypeStr=Inherit: Inherit via internal rule
  Dot Product1 : DotProduct  InputSameDT=on  OutDataTypeStr=Inherit: Inherit via internal rule
  Gain : Gain  Gain=constants.REq^3*constants.H0
  Gain1 : Gain  Gain=3
  Normalize Vector : vrlib/Utilities/Normalize Vector  maxzero=0
  Power : Math  Operator=pow  SaturateOnIntegerOverflow=on
  Product : Product
  Product1 : Product
  Sqrt : Sqrt  SaturateOnIntegerOverflow=on
  Sum : Sum  Inputs=-+
  b_n : Outport
  wires:
  rrSc_n/1 -> Normalize Vector/1, Dot Product/2, Dot Product/1
  Constant/1 -> Power/2
  Dot Product/1 -> Sqrt/1
  Sqrt/1 -> Power/1
  Power/1 -> Gain/1
  Normalize Vector/1 -> Product/2, Dot Product1/2
  mVersor/1 -> Sum/1, Dot Product1/1
  Dot Product1/1 -> Gain1/1
  Gain1/1 -> Product/1
  Product/1 -> Sum/2
  Sum/1 -> Product1/1
  Gain/1 -> Product1/2
  Product1/1 -> b_n/1

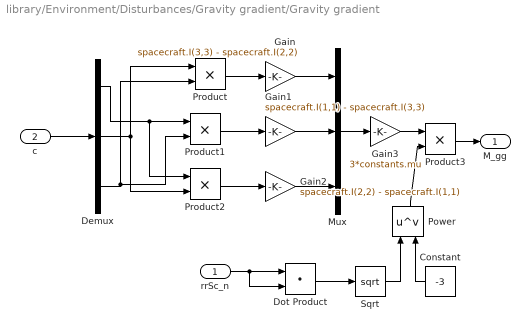
== system library/Environment/Disturbances/Gravity gradient/Gravity gradient ==
  rrSc_n : Inport
  c : Inport  Port=2
  Constant : Constant  Value=-3
  Demux : Demux  Outputs=3
  Dot Product : DotProduct  InputSameDT=on  OutDataTypeStr=Inherit: Inherit via internal rule
  Gain : Gain  Gain=spacecraft.I(3,3) - spacecraft.I(2,2)
  Gain1 : Gain  Gain=spacecraft.I(1,1) - spacecraft.I(3,3)
  Gain2 : Gain  Gain=spacecraft.I(2,2) - spacecraft.I(1,1)
  Gain3 : Gain  Gain=3*constants.mu
  Mux : Mux  Inputs=3
  Power : Math  Operator=pow  SaturateOnIntegerOverflow=on
  Product{,1..3} (4 alike) : Product
  Sqrt : Sqrt  SaturateOnIntegerOverflow=on
  M_gg : Outport
  wires:
  c/1 -> Demux/1
  Product/1 -> Gain/1
  Product1/1 -> Gain1/1
  Product2/1 -> Gain2/1
  Demux/2 -> Product2/2, Product/1
  Demux/3 -> Product1/2, Product/2
  Demux/1 -> Product2/1, Product1/1
  Gain2/1 -> Mux/3
  Gain1/1 -> Mux/2
  Gain/1 -> Mux/1
  Mux/1 -> Gain3/1
  Gain3/1 -> Product3/1
  Product3/1 -> M_gg/1
  rrSc_n/1 -> Dot Product/2, Dot Product/1
  Dot Product/1 -> Sqrt/1
  Sqrt/1 -> Power/1
  Power/1 -> Product3/2
  Constant/1 -> Power/2

== system library/Environment/Disturbances/Solar radiation pressure/SRP: active ==
  rrSc_n : Inport
  rrSun_n : Inport  Port=2
  A_bn : Inport  Port=3
  Action Port : ActionPort  ActionPortLabel=if(u1 == 1)
  Add : Sum  Inputs=-+
  Constant : Constant  Value=constants.P
  MATLAB Function : MATLAB Function  TreatAsAtomicUnit=on
  Normalize Vector : vrlib/Utilities/Normalize Vector  maxzero=0
  Product : Product  Multiplication=Matrix(*)
  Reshape : Reshape  OutputDimensionality=Column vector (2-D)
  mSRP : Outport
  vSun_n : Outport  Port=2
  wires:
  A_bn/1 -> Product/1
  rrSun_n/1 -> Add/2
  Product/1 -> Reshape/1  "vSun_b"
  Normalize Vector/1 -> vSun_n/1, Product/2
  Add/1 -> Normalize Vector/1
  MATLAB Function/1(mSRP) -> mSRP/1
  rrSc_n/1 -> Add/1
  Constant/1 -> MATLAB Function/2(P)
  Reshape/1 -> MATLAB Function/1(vSun_b)

== system library/Environment/Disturbances/Solar radiation pressure/SRP: non-active ==
  Action Port : ActionPort  ActionPortLabel=else
  Constant1 : Constant  Value=[0;0;0]
  mSRP : Outport
  wires:
  Constant1/1 -> mSRP/1

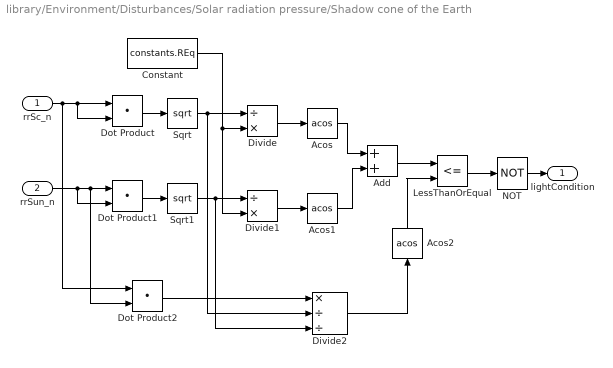
== system library/Environment/Disturbances/Solar radiation pressure/Shadow cone of the Earth ==
  rrSc_n : Inport
  rrSun_n : Inport  Port=2
  Acos : Trigonometry  Operator=acos
  Acos1 : Trigonometry  Operator=acos
  Acos2 : Trigonometry  Operator=acos
  Add : Sum
  Constant : Constant  Value=constants.REq
  Divide : Product  Inputs=/*
  Divide1 : Product  Inputs=/*
  Divide2 : Product  Inputs=*//
  Dot Product : DotProduct  InputSameDT=on  OutDataTypeStr=Inherit: Inherit via internal rule
  Dot Product1 : DotProduct  InputSameDT=on  OutDataTypeStr=Inherit: Inherit via internal rule
  Dot Product2 : DotProduct  InputSameDT=on  OutDataTypeStr=Inherit: Inherit via internal rule
  LessThanOrEqual : RelationalOperator  Operator=<=  OutDataTypeStr=boolean  RndMeth=Simplest
  NOT : Logic  Operator=NOT  IconShape=distinctive  AllPortsSameDT=off  OutDataTypeStr=boolean
  Sqrt : Sqrt  SaturateOnIntegerOverflow=on
  Sqrt1 : Sqrt  SaturateOnIntegerOverflow=on
  lightCondition : Outport
  wires:
  rrSc_n/1 -> Dot Product2/1, Dot Product/2, Dot Product/1
  Dot Product/1 -> Sqrt/1
  Dot Product1/1 -> Sqrt1/1
  rrSun_n/1 -> Dot Product1/2, Dot Product2/2, Dot Product1/1
  Sqrt/1 -> Divide2/2, Divide/1
  Sqrt1/1 -> Divide2/3, Divide1/1
  Constant/1 -> Divide1/2, Divide/2
  Divide/1 -> Acos/1
  Divide1/1 -> Acos1/1
  Dot Product2/1 -> Divide2/1
  Acos/1 -> Add/1
  Acos1/1 -> Add/2
  Add/1 -> LessThanOrEqual/1
  Divide2/1 -> Acos2/1
  LessThanOrEqual/1 -> NOT/1
  NOT/1 -> lightCondition/1
  Acos2/1 -> LessThanOrEqual/2

== system library/Environment/Disturbances/Solar radiation pressure/Sun position in the Earth inertial frame ==
  Clock : Clock
  Cos : Trigonometry  Operator=cos
  Gain : Gain  Gain=constants.nSun
  Gain1 : Gain  Gain=cos(constants.oblAngle)
  Gain2 : Gain  Gain=sin(constants.oblAngle)
  Gain3 : Gain  Gain=1*constants.AU
  Mux : Mux  Inputs=3
  Sin1 : Trigonometry
  rrSun_n : Outport
  wires:
  Gain2/1 -> Mux/3
  Clock/1 -> Gain/1
  Gain/1 -> Sin1/1, Cos/1
  Gain1/1 -> Mux/2
  Mux/1 -> Gain3/1
  Sin1/1 -> Gain2/1, Gain1/1
  Cos/1 -> Mux/1
  Gain3/1 -> rrSun_n/1

== system library/Environment/Orbit propagator/LVLH frame/LVLH to inclined orbit frame ==
  theta : Inport
  Constant : Constant  Value=0
  Constant1 : Constant  Value=[0, 0, 1]  VectorParams1D=off
  Cos : Trigonometry  Operator=cos
  Gain : Gain  Gain=-1
  Mux : Mux  Inputs=3
  Mux1 : Mux  Inputs=3
  Reshape : Reshape  OutputDimensionality=Row vector (2-D)
  Reshape1 : Reshape  OutputDimensionality=Row vector (2-D)
  Sin : Trigonometry
  Vector Concatenate : Concatenate  NumInputs=3  Mode=Multidimensional array
  A_li : Outport
  wires:
  theta/1 -> Sin/1, Cos/1
  Cos/1 -> Mux1/2, Mux/1
  Sin/1 -> Gain/1, Mux/2
  Constant/1 -> Mux1/3, Mux/3
  Gain/1 -> Mux1/1
  Mux/1 -> Reshape/1
  Constant1/1 -> Vector Concatenate/3
  Mux1/1 -> Reshape1/1
  Vector Concatenate/1 -> A_li/1
  Reshape/1 -> Vector Concatenate/1
  Reshape1/1 -> Vector Concatenate/2

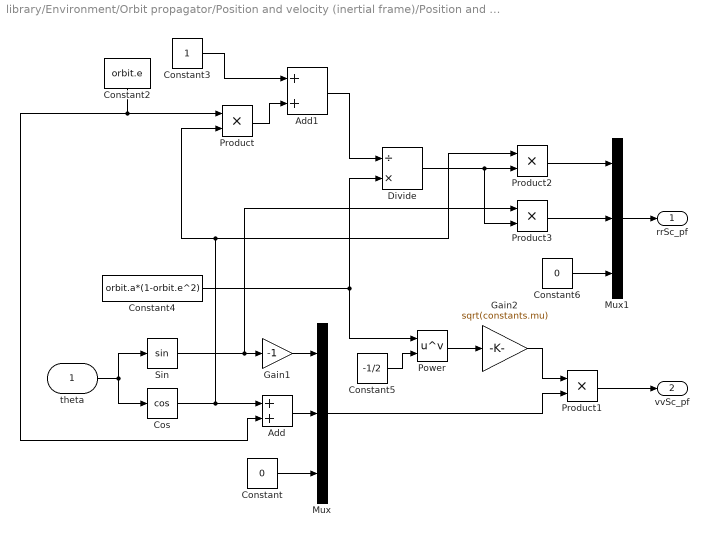
== system library/Environment/Orbit propagator/Position and velocity (inertial frame)/Position and velocity (perifocal frame) ==
  theta : Inport
  Add : Sum
  Add1 : Sum
  Constant : Constant  Value=0
  Constant2 : Constant  Value=orbit.e
  Constant3 : Constant
  Constant4 : Constant  Value=orbit.a*(1-orbit.e^2)
  Constant5 : Constant  Value=-1/2
  Constant6 : Constant  Value=0
  Cos : Trigonometry  Operator=cos
  Divide : Product  Inputs=/*
  Gain1 : Gain  Gain=-1
  Gain2 : Gain  Gain=sqrt(constants.mu)
  Mux : Mux  Inputs=3
  Mux1 : Mux  Inputs=3
  Power : Math  Operator=pow  SaturateOnIntegerOverflow=on
  Product{,1..3} (4 alike) : Product
  Sin : Trigonometry
  rrSc_pf : Outport
  vvSc_pf : Outport  Port=2
  wires:
  theta/1 -> Cos/1, Sin/1
  Mux/1 -> Product1/2
  Sin/1 -> Product3/1, Gain1/1
  Cos/1 -> Product2/1, Product/2, Add/1
  Gain1/1 -> Mux/1
  Add/1 -> Mux/2
  Constant/1 -> Mux/3
  Product1/1 -> vvSc_pf/1
  Constant3/1 -> Add1/1
  Constant2/1 -> Add/2, Product/1
  Product/1 -> Add1/2
  Add1/1 -> Divide/1
  Constant4/1 -> Divide/2, Power/1
  Constant5/1 -> Power/2
  Power/1 -> Gain2/1
  Gain2/1 -> Product1/1
  Divide/1 -> Product3/2, Product2/2
  Product2/1 -> Mux1/1
  Product3/1 -> Mux1/2
  Constant6/1 -> Mux1/3
  Mux1/1 -> rrSc_pf/1

== matlab function library/Environment/Disturbances/Solar radiation pressure/SRP: active/MATLAB Function ==
  data: vSun_b input; P input; mSRP output; surfaces parameter
function mSRP = srp(vSun_b, P, surfaces)

rSurf = surfaces.rSurf;
n = surfaces.n;
A = surfaces.A;
rhoS = surfaces.rhoS;
rhoD = surfaces.rhoD;

% Preallocation
mSRP = zeros(3,1);

% Loop on the number of surfaces
for k = 1:size(rSurf,1)
    % Extraction of the normal vector
    n_b = n(:,k);
    s_dot = dot(vSun_b, n_b);
    if s_dot > 0
        rhoS_temp = rhoS(k);
        Fsrp_i = - P*A(k)*s_dot.*((1-rhoS_temp).*vSun_b +...
            (2*rhoS_temp*s_dot + 2/3*rhoD(k)).*n_b);
        mSRP = mSRP + cross(rSurf(:,k), Fsrp_i);
    end
end

end

== matlab function library/Environment/Disturbances/Drag/MATLAB Function ==
  data: rrSc_n input; mDrag output; vvSc_n input; A_bn input; rho input; surfaces parameter
function  mDrag = drag(rrSc_n, vvSc_n, A_bn, rho, surfaces)

rSurf = surfaces.rSurf;
n = surfaces.n;
A = surfaces.A;
cd = surfaces.cd;

% Earth's angular speed
wE = 7.2921150e-5; %[rad/s]
% Relative velocity of the s/c with respect to the atmosphere
vvRel_n = [vvSc_n(1) + wE*rrSc_n(2); vvSc_n(2) - wE*rrSc_n(1); vvSc_n(3)]*1e3;
vvRel_b = A_bn*vvRel_n;

vRel_b = norm(vvRel_b);
vvVersor = vvRel_b/vRel_b;

c = -1/2*rho*cd*vRel_b^2.*vvVersor;

mDrag = zeros(3,1);

for k = 1:size(rSurf,1)
    % Extracting the normal unit vector
    n_dot = dot(n(:,k), vvVersor);
    if n_dot > 0
        A_cross = A(k)*n_dot;
        Fdrag_i = c*A_cross;
        mDrag = mDrag + cross(rSurf(:,k), Fdrag_i);
    end
end

end

== matlab function library/Attitude determination/QUEST method/Angular velocity estimation/Quaternion matrix/MATLAB Function ==
  data: Q input; Q_star output
function Q_star = pseudo_inverse(Q)

Q_star = pinv(Q);

end

== matlab function library/Attitude determination/QUEST method/MATLAB Function ==
  data: s_b input; v_n input; sensors parameter; sunInSSFoV input; estQ output; q_old input
function estQ = QUEST(s_b, v_n, sensors, sunInSSFoV, q_old)

% Definining the number of measurements
nM = size(s_b,2);

% Definining the weights based on the relative accuracies
if sunInSSFoV
    a = [1/sensors.ss.sigma; (1/sensors.st.sigma)*ones(sensors.st.nStars - 1, 1)];
else
    a = (1/sensors.st.sigma)*ones(sensors.st.nStars, 1);
end

% Normalization
a = a./sum(a);
% Preallocation
B = zeros(3);

% Filling the B matrix
for k = 1:nM
    B = B + a(k)*s_b(:,k)*v_n(:,k)';
end

% Constructing K
z = [B(2,3) - B(3,2); B(3,1) - B(1,3); B(1,2) - B(2,1)];
sigma = trace(B);
S = B + B';

K = [S - sigma*eye(3), z;...
    z', sigma];

% Solving the eigenvalue  problem and retrieving the eigenvector associated
% to lambda_max
[V, lambdaMat] = eig(K);
lambda = diag(lambdaMat);
[~, idx] = max(lambda);
q = real(V(:,idx));

% The following lines are only required in order to prevent the inversion
% of the quaternion during the simulation, as a quaternion and its negative
% physically represent the same rotation

v = abs(q - q_old);
tol = 0.1*ones(4,1);

if sum(v > tol) ~= 0
    g = -1;
else
    g = 1;
end

estQ = g*q/norm(q);

end

== matlab function library/Tracking/Ideal control law/MATLAB Function ==
  data: estAe input; lf output
function lf = linearFunction(estAe)

lf = [estAe(2,3) - estAe(3,2);...
    estAe(3,1) - estAe(1,3);...
    estAe(1,2) - estAe(2,1)];

end

== matlab function library/Attitude determination/Sensors/Magnetometer/MATLAB Function ==
  data: phi input; A_err output; theta input; psi input
function A_err = error_matrix(phi, theta, psi)

A_err = [cos(psi)*cos(theta), cos(psi)*sin(theta)*sin(phi) + sin(psi)*cos(phi),...
    -cos(psi)*sin(theta)*cos(phi) + sin(psi)*sin(phi);...
    -sin(psi)*cos(theta), -sin(psi)*sin(theta)*sin(phi) + cos(psi)*cos(phi),...
    sin(psi)*sin(theta)*cos(phi) + cos(psi)*sin(phi);...
    sin(theta), -cos(theta)*sin(phi), cos(theta)*cos(phi)];
            
end

== matlab function library/Attitude determination/Sensors/Sun sensor enabled/Star tracker/MATLAB Function ==
  data: A_bn input; s_b output; phi input; theta input; psi input; v_n_old input; v_n output; sensors parameter
function [s_b, v_n] = starTracker(A_bn, phi, theta, psi, v_n_old, sensors)

A_sb = sensors.st.A_sb;
% When the Sun sensor is working, the star tracker tracks one star less.
nStars = sensors.st.nStars - 1;
FoV = sensors.st.FoV;

A_bs = A_sb';
A_ns = A_bn'*A_bs;

% Preallocation
s_b = zeros(3,nStars); 
v_n = zeros(3,nStars);

El = zeros(nStars,1);
Az = zeros(nStars,1);

% Loop on the number of stars
for k = 0:nStars-1
    
    % Determining the position in the body and sensor frame of the star at
    % the previous time instant
    s_b_old = A_bn*v_n_old(:,end-k);
    v_s_old = A_sb*s_b_old;
    
    % Computing elevation and azimuth
    El_old = asin(v_s_old(3));
    Az_old = acos(v_s_old(1)/cos(El_old));
    
    % The azimuth shall be comprised between -pi and pi
    if v_s_old(2) <= 0
        Az_old = -Az_old;
    end
    
    % If the star is not anymore in the FoV of the sensor, a new star is
    % generated
    if abs(Az_old) > FoV(1) || abs(El_old) > FoV(2)
        Az(end-k) = 0.2*FoV(1)*(-1 + 2*rand(1,1));
        El(end-k) = 0.2*FoV(2)*(-1 + 2*rand(1,1));
        v_s = [cos(El(end-k))*cos(Az(end-k));...
            cos(El(end-k))*sin(Az(end-k));...
            sin(El(end-k))];
    else
        v_s = v_s_old;
    end
    
    % Error matrix
    A_err = [cos(psi)*cos(theta), cos(psi)*sin(theta)*sin(phi) + sin(psi)*cos(phi),...
        -cos(psi)*sin(theta)*cos(phi) + sin(psi)*sin(phi);...
        -sin(psi)*cos(theta), -sin(psi)*sin(theta)*sin(phi) + cos(psi)*cos(phi),...
        sin(psi)*sin(theta)*cos(phi) + cos(psi)*sin(phi);...
        sin(theta), -cos(theta)*sin(phi), cos(theta)*cos(phi)];
    
   % Generating the measurement (sensor and body frame)
   s_s = A_err*v_s;
   s_bTemp = A_bs*s_s;
   
   % Allocating the measurement in the measurements matrix + normalization
   s_b(1:3, end-k) = s_bTemp./norm(s_bTemp); 

   % Allocating the inertial direction in the inertial directions matrix +
   % normalization
   v_nTemp = A_ns*v_s;
   v_n(1:3,end-k) = v_nTemp;
   v_n(1:3, end-k) = v_nTemp./norm(v_nTemp);
   
end

end
